simulink model "quadrotor_mdl"  (R2021b)
settings: Solver=VariableStepAuto  StartTime=0.0  StopTime=10.0  RelTol=1e-3
settings Model: Creator=Tomo  LastModifiedBy=Tomo

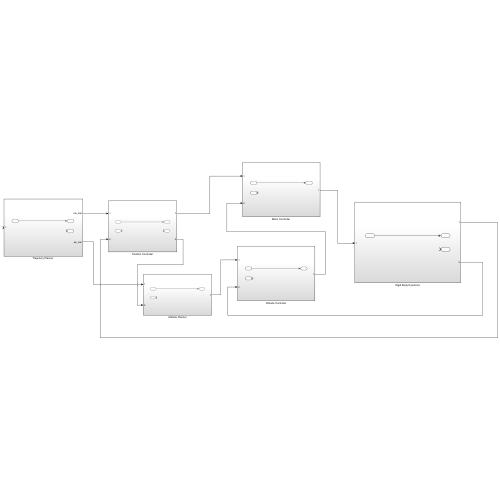
[thumbnail: Simulink's stored preview of the top-level diagram]
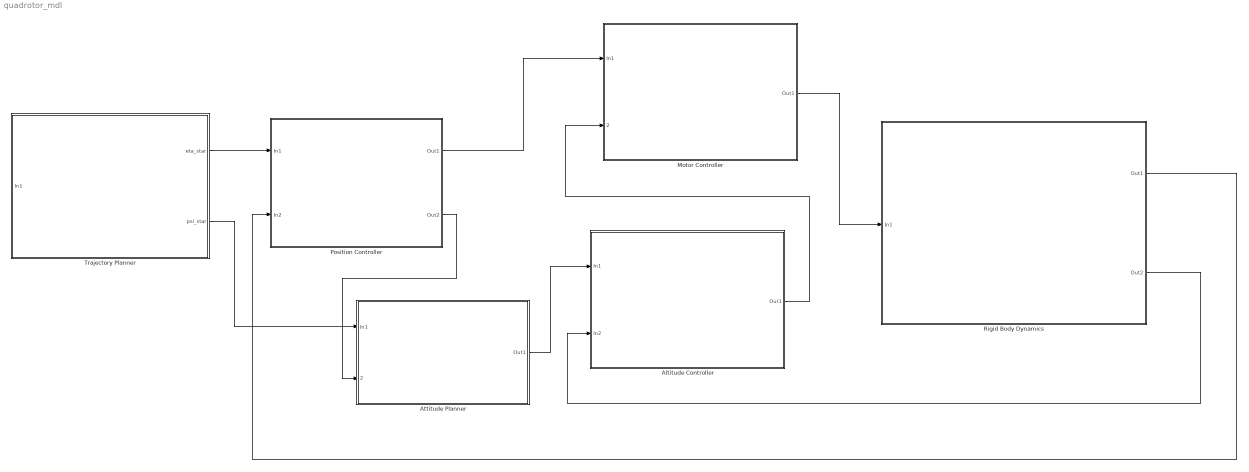
== system quadrotor_mdl ==
  Altitude Controller : Subsystem
  Attitude Planner : Subsystem
  "Motor Controller " : Subsystem
  Position Controller : Subsystem
  Rigid Body Dynamics : Subsystem
  "Trajectory Planner " : Subsystem
  wires:
  "Trajectory Planner "/1(eta_star) -> Position Controller/1(In1)
  "Trajectory Planner "/2(psi_star) -> Attitude Planner/1(In1)
  Position Controller/2(Out2) -> Attitude Planner/2(2)
  Position Controller/1(Out1) -> "Motor Controller "/1(In1)
  Attitude Planner/1(Out1) -> Altitude Controller/1(In1)
  Altitude Controller/1(Out1) -> "Motor Controller "/2(2)
  "Motor Controller "/1(Out1) -> Rigid Body Dynamics/1(In1)
  Rigid Body Dynamics/1(Out1) -> Position Controller/2(In2)
  Rigid Body Dynamics/2(Out2) -> Altitude Controller/2(In2)

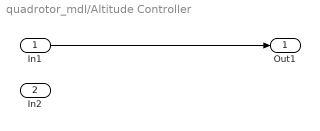
== system quadrotor_mdl/Altitude Controller ==
  In1 : Inport
  In2 : Inport  Port=2
  Out1 : Outport
  wires:
  In1/1 -> Out1/1

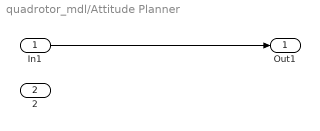
== system quadrotor_mdl/Attitude Planner ==
  In1 : Inport
  2 : Inport  Port=2
  Out1 : Outport
  wires:
  In1/1 -> Out1/1

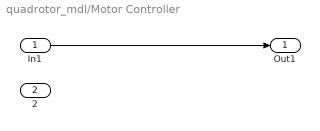
== system quadrotor_mdl/Motor Controller  ==
  In1 : Inport
  2 : Inport  Port=2
  Out1 : Outport
  wires:
  In1/1 -> Out1/1

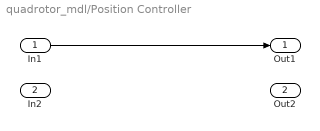
== system quadrotor_mdl/Position Controller ==
  In1 : Inport
  In2 : Inport  Port=2
  Out1 : Outport
  Out2 : Outport  Port=2
  wires:
  In1/1 -> Out1/1

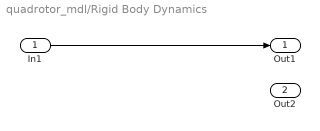
== system quadrotor_mdl/Rigid Body Dynamics ==
  In1 : Inport
  Out1 : Outport
  Out2 : Outport  Port=2
  wires:
  In1/1 -> Out1/1

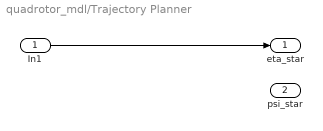
== system quadrotor_mdl/Trajectory Planner  ==
  In1 : Inport
  eta_star : Outport
  psi_star : Outport  Port=2
  wires:
  In1/1 -> eta_star/1
